simulink model "IRP"  (R2015a)
settings: Solver=ode1  StartTime=0.0  StopTime=Inf  FixedStep=0.001  RelTol=1e-3
PostLoadFcn:
  | , if any(exist('dsrtsu_mdlpostloadfcn', 'file') == [2, 3, 6]), try dsrtsu_mdlpostloadfcn('Execute', bdroot); catch fprintf('Error in PostLoadFcn (dsrtsu_mdlpostloadfcn) for model "%s":\n %s\n', bdroot, lasterr); end, end,
libraries: simulink x8, rtilibm x6, simulink_extras x6
(part 2 of 2)

== system IRP/P /Position 1/Filters 1 ==
  Sin && Cos : Inport
  Analog Butterworth LP Filter : Subsystem  mask(buttap){}
      mask help:
      | Analog Butterworth low pass filter.
      |
      | (Requires Signal Processing Toolbox)
      mask init:
      | [z,p,k]=buttap(@2); z=@1*z; p=@1*p; k=real(prod(-p)); [num,den]=zp2tf(z,p,k); w=logspace(log10(@1/10),log10(10*@1),20); h=freqs(num,den,w);
      mask Help: Butterworth low pass filter using MATLAB's butter command.
      mask Display: plot(20*log10(w),20*log10(abs(h)))
  Analog Butterworth LP Filter1 : Subsystem  mask(buttap){}
      mask help:
      | Analog Butterworth low pass filter.
      |
      | (Requires Signal Processing Toolbox)
      mask init:
      | [z,p,k]=buttap(@2); z=@1*z; p=@1*p; k=real(prod(-p)); [num,den]=zp2tf(z,p,k); w=logspace(log10(@1/10),log10(10*@1),20); h=freqs(num,den,w);
      mask Help: Butterworth low pass filter using MATLAB's butter command.
      mask Display: plot(20*log10(w),20*log10(abs(h)))
  Demux : Demux  Outputs=2
  Sin : Outport
  Cos : Outport  Port=2
  wires:
  Analog Butterworth LP Filter/1(Out1) -> Sin/1
  Analog Butterworth LP Filter1/1(Out1) -> Cos/1
  Sin && Cos/1 -> Demux/1
  Demux/1 -> Analog Butterworth LP Filter/1(In1)
  Demux/2 -> Analog Butterworth LP Filter1/1(In1)

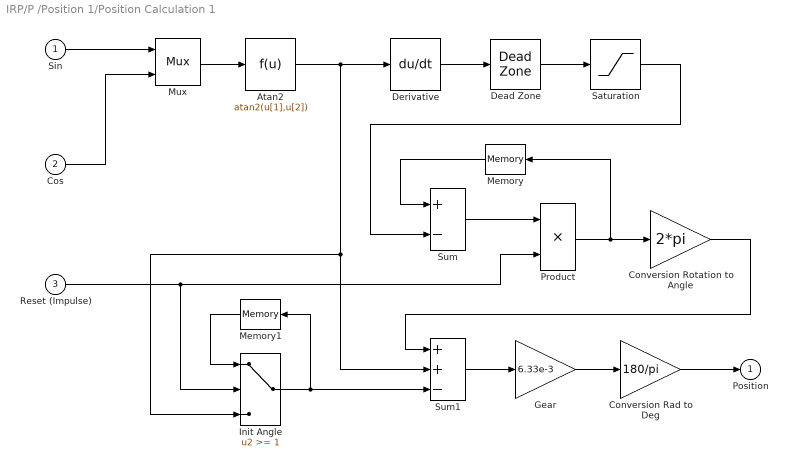
== system IRP/P /Position 1/Position Calculation 1 ==
  Sin : Inport
  Cos : Inport  Port=2
  Reset (Impulse) : Inport  Port=3
  Atan2 : Fcn  Expr=atan2(u[1],u[2])
  Conversion Rad to Deg : Gain  Gain=180/pi  SaturateOnIntegerOverflow=on  OutDataTypeStr=Inherit: Same as input  ParamDataTypeStr=Inherit: Same as input
  Conversion Rotation to Angle : Gain  Gain=2*pi  SaturateOnIntegerOverflow=on  OutDataTypeStr=Inherit: Same as input  ParamDataTypeStr=Inherit: Same as input
  Dead Zone : DeadZone  LowerValue=-5000  UpperValue=5000  SaturateOnIntegerOverflow=on
  Derivative : Derivative
  Gear : Gain  Gain=6.33e-3  SaturateOnIntegerOverflow=on  OutDataTypeStr=Inherit: Same as input  ParamDataTypeStr=Inherit: Same as input
  Init Angle : Switch  Threshold=1  SaturateOnIntegerOverflow=on  InputSameDT=on
  Memory : Memory
  Memory1 : Memory
  Mux : Mux  Inputs=2
  Product : Product  SaturateOnIntegerOverflow=on  RndMeth=Zero  InputSameDT=on  OutDataTypeStr=Inherit: Same as first input
  Saturation : Saturate  UpperLimit=1  LowerLimit=-1
  Sum : Sum  Inputs=+-  SaturateOnIntegerOverflow=on  InputSameDT=on  OutDataTypeStr=Inherit: Same as first input
  Sum1 : Sum  Inputs=++-  SaturateOnIntegerOverflow=on  InputSameDT=on  OutDataTypeStr=Inherit: Same as first input
  Position : Outport
  wires:
  Gear/1 -> Conversion Rad to Deg/1
  Sum1/1 -> Gear/1
  Sum/1 -> Product/1
  Dead Zone/1 -> Saturation/1
  Derivative/1 -> Dead Zone/1
  Mux/1 -> Atan2/1
  Sin/1 -> Mux/1
  Conversion Rad to Deg/1 -> Position/1
  Saturation/1 -> Sum/2
  Conversion Rotation to Angle/1 -> Sum1/1
  Reset (Impulse)/1 -> Product/2, Init Angle/2
  Atan2/1 -> Derivative/1, Sum1/2, Init Angle/3
  Cos/1 -> Mux/2
  Memory/1 -> Sum/1
  Product/1 -> Conversion Rotation to Angle/1, Memory/1
  Memory1/1 -> Init Angle/1
  Init Angle/1 -> Sum1/3, Memory1/1

== system IRP/P /Position 2/Filters 2 ==
  Sin && Cos : Inport
  Analog Butterworth LP Filter : Subsystem  mask(buttap){}
      mask help:
      | Analog Butterworth low pass filter.
      |
      | (Requires Signal Processing Toolbox)
      mask init:
      | [z,p,k]=buttap(@2); z=@1*z; p=@1*p; k=real(prod(-p)); [num,den]=zp2tf(z,p,k); w=logspace(log10(@1/10),log10(10*@1),20); h=freqs(num,den,w);
      mask Help: Butterworth low pass filter using MATLAB's butter command.
      mask Display: plot(20*log10(w),20*log10(abs(h)))
  Analog Butterworth LP Filter1 : Subsystem  mask(buttap){}
      mask help:
      | Analog Butterworth low pass filter.
      |
      | (Requires Signal Processing Toolbox)
      mask init:
      | [z,p,k]=buttap(@2); z=@1*z; p=@1*p; k=real(prod(-p)); [num,den]=zp2tf(z,p,k); w=logspace(log10(@1/10),log10(10*@1),20); h=freqs(num,den,w);
      mask Help: Butterworth low pass filter using MATLAB's butter command.
      mask Display: plot(20*log10(w),20*log10(abs(h)))
  Demux : Demux  Outputs=2
  Sin : Outport
  Cos : Outport  Port=2
  wires:
  Analog Butterworth LP Filter/1(Out1) -> Sin/1
  Analog Butterworth LP Filter1/1(Out1) -> Cos/1
  Sin && Cos/1 -> Demux/1
  Demux/1 -> Analog Butterworth LP Filter/1(In1)
  Demux/2 -> Analog Butterworth LP Filter1/1(In1)

== system IRP/P /Position 2/Position Calculation 2 ==
  Sin : Inport
  Cos : Inport  Port=2
  Reset (Impulse) : Inport  Port=3
  Atan2 : Fcn  Expr=atan2(u[1],u[2])
  Conversion Rad to Deg : Gain  Gain=180/pi  SaturateOnIntegerOverflow=on  OutDataTypeStr=Inherit: Same as input  ParamDataTypeStr=Inherit: Same as input
  Conversion Rotation to Angle : Gain  Gain=2*pi  SaturateOnIntegerOverflow=on  OutDataTypeStr=Inherit: Same as input  ParamDataTypeStr=Inherit: Same as input
  Dead Zone : DeadZone  LowerValue=-5000  UpperValue=5000  SaturateOnIntegerOverflow=on
  Derivative : Derivative
  Gear : Gain  Gain=6.37e-3  SaturateOnIntegerOverflow=on  OutDataTypeStr=Inherit: Same as input  ParamDataTypeStr=Inherit: Same as input
  Init Angle : Switch  Threshold=1  SaturateOnIntegerOverflow=on  InputSameDT=on
  Memory : Memory
  Memory1 : Memory
  Mux : Mux  Inputs=2
  Product : Product  SaturateOnIntegerOverflow=on  RndMeth=Zero  InputSameDT=on  OutDataTypeStr=Inherit: Same as first input
  Saturation : Saturate  UpperLimit=1  LowerLimit=-1
  Sum : Sum  Inputs=+-  SaturateOnIntegerOverflow=on  InputSameDT=on  OutDataTypeStr=Inherit: Same as first input
  Sum1 : Sum  Inputs=++-  SaturateOnIntegerOverflow=on  InputSameDT=on  OutDataTypeStr=Inherit: Same as first input
  Position : Outport
  wires:
  Gear/1 -> Conversion Rad to Deg/1
  Sum1/1 -> Gear/1
  Sum/1 -> Product/1
  Dead Zone/1 -> Saturation/1
  Derivative/1 -> Dead Zone/1
  Mux/1 -> Atan2/1
  Sin/1 -> Mux/1
  Conversion Rad to Deg/1 -> Position/1
  Saturation/1 -> Sum/2
  Conversion Rotation to Angle/1 -> Sum1/1
  Reset (Impulse)/1 -> Product/2, Init Angle/2
  Atan2/1 -> Derivative/1, Sum1/2, Init Angle/3
  Cos/1 -> Mux/2
  Memory/1 -> Sum/1
  Product/1 -> Conversion Rotation to Angle/1, Memory/1
  Memory1/1 -> Init Angle/1
  Init Angle/1 -> Sum1/3, Memory1/1

== system IRP/P /Position 3/Filters 3 ==
  Sin && Cos : Inport
  Analog Butterworth LP Filter : Subsystem  mask(buttap){}
      mask help:
      | Analog Butterworth low pass filter.
      |
      | (Requires Signal Processing Toolbox)
      mask init:
      | [z,p,k]=buttap(@2); z=@1*z; p=@1*p; k=real(prod(-p)); [num,den]=zp2tf(z,p,k); w=logspace(log10(@1/10),log10(10*@1),20); h=freqs(num,den,w);
      mask Help: Butterworth low pass filter using MATLAB's butter command.
      mask Display: plot(20*log10(w),20*log10(abs(h)))
  Analog Butterworth LP Filter1 : Subsystem  mask(buttap){}
      mask help:
      | Analog Butterworth low pass filter.
      |
      | (Requires Signal Processing Toolbox)
      mask init:
      | [z,p,k]=buttap(@2); z=@1*z; p=@1*p; k=real(prod(-p)); [num,den]=zp2tf(z,p,k); w=logspace(log10(@1/10),log10(10*@1),20); h=freqs(num,den,w);
      mask Help: Butterworth low pass filter using MATLAB's butter command.
      mask Display: plot(20*log10(w),20*log10(abs(h)))
  Demux : Demux  Outputs=2
  Sin : Outport
  Cos : Outport  Port=2
  wires:
  Analog Butterworth LP Filter/1(Out1) -> Sin/1
  Analog Butterworth LP Filter1/1(Out1) -> Cos/1
  Sin && Cos/1 -> Demux/1
  Demux/1 -> Analog Butterworth LP Filter/1(In1)
  Demux/2 -> Analog Butterworth LP Filter1/1(In1)

== system IRP/P /Position 3/Position Calculation 3 ==
  Sin : Inport
  Cos : Inport  Port=2
  Reset (Impulse) : Inport  Port=3
  Atan2 : Fcn  Expr=atan2(u[1],u[2])
  Conversion Rad to Deg : Gain  Gain=180/pi  SaturateOnIntegerOverflow=on  OutDataTypeStr=Inherit: Same as input  ParamDataTypeStr=Inherit: Same as input
  Conversion Rotation to Angle : Gain  Gain=2*pi  SaturateOnIntegerOverflow=on  OutDataTypeStr=Inherit: Same as input  ParamDataTypeStr=Inherit: Same as input
  Dead Zone : DeadZone  LowerValue=-5000  UpperValue=5000  SaturateOnIntegerOverflow=on
  Derivative : Derivative
  Gear : Gain  Gain=6.33e-3  SaturateOnIntegerOverflow=on  OutDataTypeStr=Inherit: Same as input  ParamDataTypeStr=Inherit: Same as input
  Init Angle : Switch  Threshold=1  SaturateOnIntegerOverflow=on  InputSameDT=on
  Memory : Memory
  Memory1 : Memory
  Mux : Mux  Inputs=2
  Product : Product  SaturateOnIntegerOverflow=on  RndMeth=Zero  InputSameDT=on  OutDataTypeStr=Inherit: Same as first input
  Saturation : Saturate  UpperLimit=1  LowerLimit=-1
  Sum : Sum  Inputs=+-  SaturateOnIntegerOverflow=on  InputSameDT=on  OutDataTypeStr=Inherit: Same as first input
  Sum1 : Sum  Inputs=++-  SaturateOnIntegerOverflow=on  InputSameDT=on  OutDataTypeStr=Inherit: Same as first input
  Position : Outport
  wires:
  Gear/1 -> Conversion Rad to Deg/1
  Sum1/1 -> Gear/1
  Sum/1 -> Product/1
  Dead Zone/1 -> Saturation/1
  Derivative/1 -> Dead Zone/1
  Mux/1 -> Atan2/1
  Sin/1 -> Mux/1
  Conversion Rad to Deg/1 -> Position/1
  Saturation/1 -> Sum/2
  Conversion Rotation to Angle/1 -> Sum1/1
  Reset (Impulse)/1 -> Product/2, Init Angle/2
  Atan2/1 -> Derivative/1, Sum1/2, Init Angle/3
  Cos/1 -> Mux/2
  Memory/1 -> Sum/1
  Product/1 -> Conversion Rotation to Angle/1, Memory/1
  Memory1/1 -> Init Angle/1
  Init Angle/1 -> Sum1/3, Memory1/1

== system IRP/P /Position 4/Filters 4 ==
  Sin && Cos : Inport
  Analog Butterworth LP Filter : Subsystem  mask(buttap){}
      mask help:
      | Analog Butterworth low pass filter.
      |
      | (Requires Signal Processing Toolbox)
      mask init:
      | [z,p,k]=buttap(@2); z=@1*z; p=@1*p; k=real(prod(-p)); [num,den]=zp2tf(z,p,k); w=logspace(log10(@1/10),log10(10*@1),20); h=freqs(num,den,w);
      mask Help: Butterworth low pass filter using MATLAB's butter command.
      mask Display: plot(20*log10(w),20*log10(abs(h)))
  Analog Butterworth LP Filter1 : Subsystem  mask(buttap){}
      mask help:
      | Analog Butterworth low pass filter.
      |
      | (Requires Signal Processing Toolbox)
      mask init:
      | [z,p,k]=buttap(@2); z=@1*z; p=@1*p; k=real(prod(-p)); [num,den]=zp2tf(z,p,k); w=logspace(log10(@1/10),log10(10*@1),20); h=freqs(num,den,w);
      mask Help: Butterworth low pass filter using MATLAB's butter command.
      mask Display: plot(20*log10(w),20*log10(abs(h)))
  Demux : Demux  Outputs=2
  Sin : Outport
  Cos : Outport  Port=2
  wires:
  Demux/2 -> Analog Butterworth LP Filter1/1(In1)
  Demux/1 -> Analog Butterworth LP Filter/1(In1)
  Sin && Cos/1 -> Demux/1
  Analog Butterworth LP Filter1/1(Out1) -> Cos/1
  Analog Butterworth LP Filter/1(Out1) -> Sin/1

== system IRP/P /Position 4/Position Calculation 4 ==
  Sin : Inport
  Cos : Inport  Port=2
  Reset (Impulse) : Inport  Port=3
  Atan2 : Fcn  Expr=atan2(u[1],u[2])
  Conversion Rad to Deg : Gain  Gain=180/pi  SaturateOnIntegerOverflow=on  OutDataTypeStr=Inherit: Same as input  ParamDataTypeStr=Inherit: Same as input
  Conversion Rotation to Angle : Gain  Gain=2*pi  SaturateOnIntegerOverflow=on  OutDataTypeStr=Inherit: Same as input  ParamDataTypeStr=Inherit: Same as input
  Dead Zone : DeadZone  LowerValue=-5000  UpperValue=5000  SaturateOnIntegerOverflow=on
  Derivative : Derivative
  Gear : Gain  Gain=7.87e-3  SaturateOnIntegerOverflow=on  OutDataTypeStr=Inherit: Same as input  ParamDataTypeStr=Inherit: Same as input
  Init Angle : Switch  Threshold=1  SaturateOnIntegerOverflow=on  InputSameDT=on
  Memory : Memory
  Memory1 : Memory
  Mux : Mux  Inputs=2
  Product : Product  SaturateOnIntegerOverflow=on  RndMeth=Zero  InputSameDT=on  OutDataTypeStr=Inherit: Same as first input
  Saturation : Saturate  UpperLimit=1  LowerLimit=-1
  Sum : Sum  Inputs=+-  SaturateOnIntegerOverflow=on  InputSameDT=on  OutDataTypeStr=Inherit: Same as first input
  Sum1 : Sum  Inputs=++-  SaturateOnIntegerOverflow=on  InputSameDT=on  OutDataTypeStr=Inherit: Same as first input
  Position : Outport
  wires:
  Init Angle/1 -> Memory1/1, Sum1/3
  Memory1/1 -> Init Angle/1
  Product/1 -> Memory/1, Conversion Rotation to Angle/1
  Memory/1 -> Sum/1
  Cos/1 -> Mux/2
  Atan2/1 -> Init Angle/3, Sum1/2, Derivative/1
  Reset (Impulse)/1 -> Init Angle/2, Product/2
  Conversion Rotation to Angle/1 -> Sum1/1
  Saturation/1 -> Sum/2
  Conversion Rad to Deg/1 -> Position/1
  Sin/1 -> Mux/1
  Mux/1 -> Atan2/1
  Derivative/1 -> Dead Zone/1
  Dead Zone/1 -> Saturation/1
  Sum/1 -> Product/1
  Sum1/1 -> Gear/1
  Gear/1 -> Conversion Rad to Deg/1

== system IRP/P /Position 5/Filters 5 ==
  Sin && Cos : Inport
  Analog Butterworth LP Filter : Subsystem  mask(buttap){}
      mask help:
      | Analog Butterworth low pass filter.
      |
      | (Requires Signal Processing Toolbox)
      mask init:
      | [z,p,k]=buttap(@2); z=@1*z; p=@1*p; k=real(prod(-p)); [num,den]=zp2tf(z,p,k); w=logspace(log10(@1/10),log10(10*@1),20); h=freqs(num,den,w);
      mask Help: Butterworth low pass filter using MATLAB's butter command.
      mask Display: plot(20*log10(w),20*log10(abs(h)))
  Analog Butterworth LP Filter1 : Subsystem  mask(buttap){}
      mask help:
      | Analog Butterworth low pass filter.
      |
      | (Requires Signal Processing Toolbox)
      mask init:
      | [z,p,k]=buttap(@2); z=@1*z; p=@1*p; k=real(prod(-p)); [num,den]=zp2tf(z,p,k); w=logspace(log10(@1/10),log10(10*@1),20); h=freqs(num,den,w);
      mask Help: Butterworth low pass filter using MATLAB's butter command.
      mask Display: plot(20*log10(w),20*log10(abs(h)))
  Demux : Demux  Outputs=2
  Sin : Outport
  Cos : Outport  Port=2
  wires:
  Demux/2 -> Analog Butterworth LP Filter1/1(In1)
  Demux/1 -> Analog Butterworth LP Filter/1(In1)
  Sin && Cos/1 -> Demux/1
  Analog Butterworth LP Filter1/1(Out1) -> Cos/1
  Analog Butterworth LP Filter/1(Out1) -> Sin/1

== system IRP/P /Position 5/Position Calculation 5 ==
  Sin : Inport
  Cos : Inport  Port=2
  Reset (Impulse) : Inport  Port=3
  Atan2 : Fcn  Expr=atan2(u[1],u[2])
  Conversion Rad to Deg : Gain  Gain=180/pi  SaturateOnIntegerOverflow=on  OutDataTypeStr=Inherit: Same as input  ParamDataTypeStr=Inherit: Same as input
  Conversion Rotation to Angle : Gain  Gain=2*pi  SaturateOnIntegerOverflow=on  OutDataTypeStr=Inherit: Same as input  ParamDataTypeStr=Inherit: Same as input
  Dead Zone : DeadZone  LowerValue=-5000  UpperValue=5000  SaturateOnIntegerOverflow=on
  Derivative : Derivative
  Gear : Gain  Gain=1.32e-2  SaturateOnIntegerOverflow=on  OutDataTypeStr=Inherit: Same as input  ParamDataTypeStr=Inherit: Same as input
  Init Angle : Switch  Threshold=1  SaturateOnIntegerOverflow=on  InputSameDT=on
  Memory : Memory
  Memory1 : Memory
  Mux : Mux  Inputs=2
  Product : Product  SaturateOnIntegerOverflow=on  RndMeth=Zero  InputSameDT=on  OutDataTypeStr=Inherit: Same as first input
  Saturation : Saturate  UpperLimit=1  LowerLimit=-1
  Sum : Sum  Inputs=+-  SaturateOnIntegerOverflow=on  InputSameDT=on  OutDataTypeStr=Inherit: Same as first input
  Sum1 : Sum  Inputs=++-  SaturateOnIntegerOverflow=on  InputSameDT=on  OutDataTypeStr=Inherit: Same as first input
  Position : Outport
  wires:
  Init Angle/1 -> Memory1/1, Sum1/3
  Memory1/1 -> Init Angle/1
  Product/1 -> Memory/1, Conversion Rotation to Angle/1
  Memory/1 -> Sum/1
  Cos/1 -> Mux/2
  Atan2/1 -> Init Angle/3, Sum1/2, Derivative/1
  Reset (Impulse)/1 -> Init Angle/2, Product/2
  Conversion Rotation to Angle/1 -> Sum1/1
  Saturation/1 -> Sum/2
  Conversion Rad to Deg/1 -> Position/1
  Sin/1 -> Mux/1
  Mux/1 -> Atan2/1
  Derivative/1 -> Dead Zone/1
  Dead Zone/1 -> Saturation/1
  Sum/1 -> Product/1
  Sum1/1 -> Gear/1
  Gear/1 -> Conversion Rad to Deg/1

== system IRP/RTI Data/RTI Data Store/RTI Data Store ==
  RTI Data Store : Subsystem  mask(RTI_DATA_STORE){}
      mask help:
      | RTI Data Store Block. This block is used by RTI to store internal model dependent data. Deleting this block will result in data loss.
      |
      | NEVER DELETE, COPY, OR MODIFY THIS BLOCK!
      mask Help:
      | RTI Data Store Block. This block is used by RTI to store internal model dependent data. Deleting this block will result in data loss.
      | 
      | NEVER DELETE, COPY, OR MODIFY THIS BLOCK!
      mask Display: text(0.5, 0.5, ' ', 'HorizontalAlignment', 'center');

== system IRP/Const/Subsystem/Position 1/Filters 1 ==
  Sin && Cos : Inport
  Analog Butterworth LP Filter : Subsystem  mask(buttap){}
      mask help:
      | Analog Butterworth low pass filter.
      |
      | (Requires Signal Processing Toolbox)
      mask init:
      | [z,p,k]=buttap(@2); z=@1*z; p=@1*p; k=real(prod(-p)); [num,den]=zp2tf(z,p,k); w=logspace(log10(@1/10),log10(10*@1),20); h=freqs(num,den,w);
      mask Help: Butterworth low pass filter using MATLAB's butter command.
      mask Display: plot(20*log10(w),20*log10(abs(h)))
  Analog Butterworth LP Filter1 : Subsystem  mask(buttap){}
      mask help:
      | Analog Butterworth low pass filter.
      |
      | (Requires Signal Processing Toolbox)
      mask init:
      | [z,p,k]=buttap(@2); z=@1*z; p=@1*p; k=real(prod(-p)); [num,den]=zp2tf(z,p,k); w=logspace(log10(@1/10),log10(10*@1),20); h=freqs(num,den,w);
      mask Help: Butterworth low pass filter using MATLAB's butter command.
      mask Display: plot(20*log10(w),20*log10(abs(h)))
  Demux : Demux  Outputs=2
  Sin : Outport
  Cos : Outport  Port=2
  wires:
  Analog Butterworth LP Filter/1(Out1) -> Sin/1
  Analog Butterworth LP Filter1/1(Out1) -> Cos/1
  Sin && Cos/1 -> Demux/1
  Demux/1 -> Analog Butterworth LP Filter/1(In1)
  Demux/2 -> Analog Butterworth LP Filter1/1(In1)

== system IRP/Const/Subsystem/Position 1/Position Calculation 1 ==
  Sin : Inport
  Cos : Inport  Port=2
  Reset (Impulse) : Inport  Port=3
  Atan2 : Fcn  Expr=atan2(u[1],u[2])
  Conversion Rad to Deg : Gain  Gain=180/pi  SaturateOnIntegerOverflow=on  OutDataTypeStr=Inherit: Same as input  ParamDataTypeStr=Inherit: Same as input
  Conversion Rotation to Angle : Gain  Gain=2*pi  SaturateOnIntegerOverflow=on  OutDataTypeStr=Inherit: Same as input  ParamDataTypeStr=Inherit: Same as input
  Dead Zone : DeadZone  LowerValue=-5000  UpperValue=5000  SaturateOnIntegerOverflow=on
  Derivative : Derivative
  Gear : Gain  Gain=6.33e-3  SaturateOnIntegerOverflow=on  OutDataTypeStr=Inherit: Same as input  ParamDataTypeStr=Inherit: Same as input
  Init Angle : Switch  Threshold=1  SaturateOnIntegerOverflow=on  InputSameDT=on
  Memory : Memory
  Memory1 : Memory
  Mux : Mux  Inputs=2
  Product : Product  SaturateOnIntegerOverflow=on  RndMeth=Zero  InputSameDT=on  OutDataTypeStr=Inherit: Same as first input
  Saturation : Saturate  UpperLimit=1  LowerLimit=-1
  Sum : Sum  Inputs=+-  SaturateOnIntegerOverflow=on  InputSameDT=on  OutDataTypeStr=Inherit: Same as first input
  Sum1 : Sum  Inputs=++-  SaturateOnIntegerOverflow=on  InputSameDT=on  OutDataTypeStr=Inherit: Same as first input
  Position : Outport
  wires:
  Gear/1 -> Conversion Rad to Deg/1
  Sum1/1 -> Gear/1
  Sum/1 -> Product/1
  Dead Zone/1 -> Saturation/1
  Derivative/1 -> Dead Zone/1
  Mux/1 -> Atan2/1
  Sin/1 -> Mux/1
  Conversion Rad to Deg/1 -> Position/1
  Saturation/1 -> Sum/2
  Conversion Rotation to Angle/1 -> Sum1/1
  Reset (Impulse)/1 -> Product/2, Init Angle/2
  Atan2/1 -> Derivative/1, Sum1/2, Init Angle/3
  Cos/1 -> Mux/2
  Memory/1 -> Sum/1
  Product/1 -> Conversion Rotation to Angle/1, Memory/1
  Memory1/1 -> Init Angle/1
  Init Angle/1 -> Sum1/3, Memory1/1

== system IRP/Const/Subsystem/Position 2/Filters 2 ==
  Sin && Cos : Inport
  Analog Butterworth LP Filter : Subsystem  mask(buttap){}
      mask help:
      | Analog Butterworth low pass filter.
      |
      | (Requires Signal Processing Toolbox)
      mask init:
      | [z,p,k]=buttap(@2); z=@1*z; p=@1*p; k=real(prod(-p)); [num,den]=zp2tf(z,p,k); w=logspace(log10(@1/10),log10(10*@1),20); h=freqs(num,den,w);
      mask Help: Butterworth low pass filter using MATLAB's butter command.
      mask Display: plot(20*log10(w),20*log10(abs(h)))
  Analog Butterworth LP Filter1 : Subsystem  mask(buttap){}
      mask help:
      | Analog Butterworth low pass filter.
      |
      | (Requires Signal Processing Toolbox)
      mask init:
      | [z,p,k]=buttap(@2); z=@1*z; p=@1*p; k=real(prod(-p)); [num,den]=zp2tf(z,p,k); w=logspace(log10(@1/10),log10(10*@1),20); h=freqs(num,den,w);
      mask Help: Butterworth low pass filter using MATLAB's butter command.
      mask Display: plot(20*log10(w),20*log10(abs(h)))
  Demux : Demux  Outputs=2
  Sin : Outport
  Cos : Outport  Port=2
  wires:
  Analog Butterworth LP Filter/1(Out1) -> Sin/1
  Analog Butterworth LP Filter1/1(Out1) -> Cos/1
  Sin && Cos/1 -> Demux/1
  Demux/1 -> Analog Butterworth LP Filter/1(In1)
  Demux/2 -> Analog Butterworth LP Filter1/1(In1)

== system IRP/Const/Subsystem/Position 2/Position Calculation 2 ==
  Sin : Inport
  Cos : Inport  Port=2
  Reset (Impulse) : Inport  Port=3
  Atan2 : Fcn  Expr=atan2(u[1],u[2])
  Conversion Rad to Deg : Gain  Gain=180/pi  SaturateOnIntegerOverflow=on  OutDataTypeStr=Inherit: Same as input  ParamDataTypeStr=Inherit: Same as input
  Conversion Rotation to Angle : Gain  Gain=2*pi  SaturateOnIntegerOverflow=on  OutDataTypeStr=Inherit: Same as input  ParamDataTypeStr=Inherit: Same as input
  Dead Zone : DeadZone  LowerValue=-5000  UpperValue=5000  SaturateOnIntegerOverflow=on
  Derivative : Derivative
  Gear : Gain  Gain=6.37e-3  SaturateOnIntegerOverflow=on  OutDataTypeStr=Inherit: Same as input  ParamDataTypeStr=Inherit: Same as input
  Init Angle : Switch  Threshold=1  SaturateOnIntegerOverflow=on  InputSameDT=on
  Memory : Memory
  Memory1 : Memory
  Mux : Mux  Inputs=2
  Product : Product  SaturateOnIntegerOverflow=on  RndMeth=Zero  InputSameDT=on  OutDataTypeStr=Inherit: Same as first input
  Saturation : Saturate  UpperLimit=1  LowerLimit=-1
  Sum : Sum  Inputs=+-  SaturateOnIntegerOverflow=on  InputSameDT=on  OutDataTypeStr=Inherit: Same as first input
  Sum1 : Sum  Inputs=++-  SaturateOnIntegerOverflow=on  InputSameDT=on  OutDataTypeStr=Inherit: Same as first input
  Position : Outport
  wires:
  Gear/1 -> Conversion Rad to Deg/1
  Sum1/1 -> Gear/1
  Sum/1 -> Product/1
  Dead Zone/1 -> Saturation/1
  Derivative/1 -> Dead Zone/1
  Mux/1 -> Atan2/1
  Sin/1 -> Mux/1
  Conversion Rad to Deg/1 -> Position/1
  Saturation/1 -> Sum/2
  Conversion Rotation to Angle/1 -> Sum1/1
  Reset (Impulse)/1 -> Product/2, Init Angle/2
  Atan2/1 -> Derivative/1, Sum1/2, Init Angle/3
  Cos/1 -> Mux/2
  Memory/1 -> Sum/1
  Product/1 -> Conversion Rotation to Angle/1, Memory/1
  Memory1/1 -> Init Angle/1
  Init Angle/1 -> Sum1/3, Memory1/1

== system IRP/Const/Subsystem/Position 3/Filters 3 ==
  Sin && Cos : Inport
  Analog Butterworth LP Filter : Subsystem  mask(buttap){}
      mask help:
      | Analog Butterworth low pass filter.
      |
      | (Requires Signal Processing Toolbox)
      mask init:
      | [z,p,k]=buttap(@2); z=@1*z; p=@1*p; k=real(prod(-p)); [num,den]=zp2tf(z,p,k); w=logspace(log10(@1/10),log10(10*@1),20); h=freqs(num,den,w);
      mask Help: Butterworth low pass filter using MATLAB's butter command.
      mask Display: plot(20*log10(w),20*log10(abs(h)))
  Analog Butterworth LP Filter1 : Subsystem  mask(buttap){}
      mask help:
      | Analog Butterworth low pass filter.
      |
      | (Requires Signal Processing Toolbox)
      mask init:
      | [z,p,k]=buttap(@2); z=@1*z; p=@1*p; k=real(prod(-p)); [num,den]=zp2tf(z,p,k); w=logspace(log10(@1/10),log10(10*@1),20); h=freqs(num,den,w);
      mask Help: Butterworth low pass filter using MATLAB's butter command.
      mask Display: plot(20*log10(w),20*log10(abs(h)))
  Demux : Demux  Outputs=2
  Sin : Outport
  Cos : Outport  Port=2
  wires:
  Analog Butterworth LP Filter/1(Out1) -> Sin/1
  Analog Butterworth LP Filter1/1(Out1) -> Cos/1
  Sin && Cos/1 -> Demux/1
  Demux/1 -> Analog Butterworth LP Filter/1(In1)
  Demux/2 -> Analog Butterworth LP Filter1/1(In1)

== system IRP/Const/Subsystem/Position 3/Position Calculation 3 ==
  Sin : Inport
  Cos : Inport  Port=2
  Reset (Impulse) : Inport  Port=3
  Atan2 : Fcn  Expr=atan2(u[1],u[2])
  Conversion Rad to Deg : Gain  Gain=180/pi  SaturateOnIntegerOverflow=on  OutDataTypeStr=Inherit: Same as input  ParamDataTypeStr=Inherit: Same as input
  Conversion Rotation to Angle : Gain  Gain=2*pi  SaturateOnIntegerOverflow=on  OutDataTypeStr=Inherit: Same as input  ParamDataTypeStr=Inherit: Same as input
  Dead Zone : DeadZone  LowerValue=-5000  UpperValue=5000  SaturateOnIntegerOverflow=on
  Derivative : Derivative
  Gear : Gain  Gain=6.33e-3  SaturateOnIntegerOverflow=on  OutDataTypeStr=Inherit: Same as input  ParamDataTypeStr=Inherit: Same as input
  Init Angle : Switch  Threshold=1  SaturateOnIntegerOverflow=on  InputSameDT=on
  Memory : Memory
  Memory1 : Memory
  Mux : Mux  Inputs=2
  Product : Product  SaturateOnIntegerOverflow=on  RndMeth=Zero  InputSameDT=on  OutDataTypeStr=Inherit: Same as first input
  Saturation : Saturate  UpperLimit=1  LowerLimit=-1
  Sum : Sum  Inputs=+-  SaturateOnIntegerOverflow=on  InputSameDT=on  OutDataTypeStr=Inherit: Same as first input
  Sum1 : Sum  Inputs=++-  SaturateOnIntegerOverflow=on  InputSameDT=on  OutDataTypeStr=Inherit: Same as first input
  Position : Outport
  wires:
  Gear/1 -> Conversion Rad to Deg/1
  Sum1/1 -> Gear/1
  Sum/1 -> Product/1
  Dead Zone/1 -> Saturation/1
  Derivative/1 -> Dead Zone/1
  Mux/1 -> Atan2/1
  Sin/1 -> Mux/1
  Conversion Rad to Deg/1 -> Position/1
  Saturation/1 -> Sum/2
  Conversion Rotation to Angle/1 -> Sum1/1
  Reset (Impulse)/1 -> Product/2, Init Angle/2
  Atan2/1 -> Derivative/1, Sum1/2, Init Angle/3
  Cos/1 -> Mux/2
  Memory/1 -> Sum/1
  Product/1 -> Conversion Rotation to Angle/1, Memory/1
  Memory1/1 -> Init Angle/1
  Init Angle/1 -> Sum1/3, Memory1/1

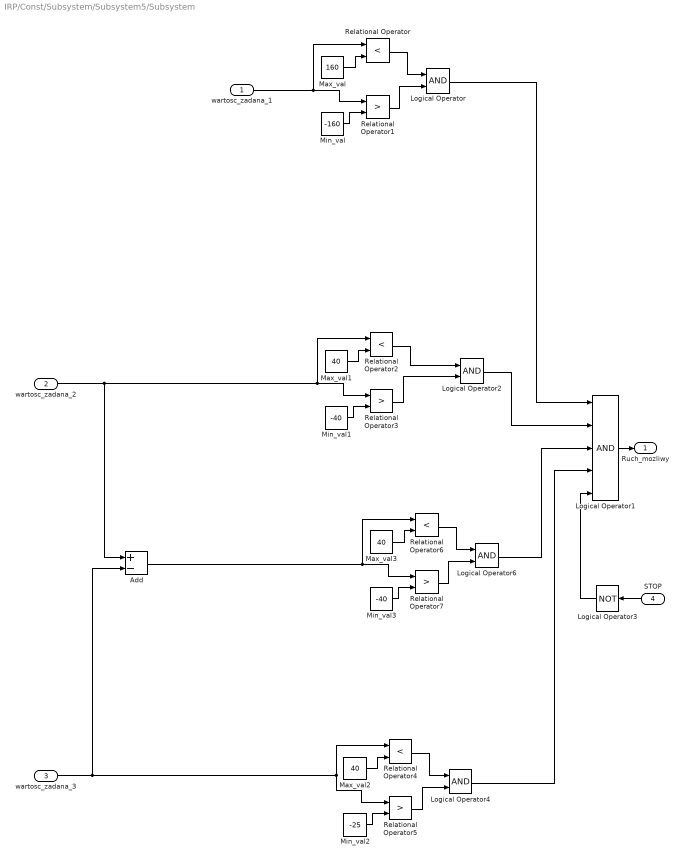
== system IRP/Const/Subsystem/Subsystem5/Subsystem ==
  wartosc_zadana_1 : Inport
  wartosc_zadana_2 : Inport  Port=2
  wartosc_zadana_3 : Inport  Port=3
  STOP : Inport  Port=4
  Add : Sum  Inputs=+-
  Logical Operator{,2,4,6} (4 alike) : Logic  AllPortsSameDT=off
  Logical Operator1 : Logic  Inputs=5  AllPortsSameDT=off
  Logical Operator3 : Logic  Operator=NOT  AllPortsSameDT=off
  Max_val : Constant  Value=160
  Max_val1 : Constant  Value=40
  Max_val2 : Constant  Value=40
  Max_val3 : Constant  Value=40
  Min_val : Constant  Value=-160
  Min_val1 : Constant  Value=-40
  Min_val2 : Constant  Value=-25
  Min_val3 : Constant  Value=-40
  Relational Operator{,2,4,6} (4 alike) : RelationalOperator  Operator=<  OutDataTypeStr=boolean
  Relational Operator{1,3,5,7} (4 alike) : RelationalOperator  Operator=>  OutDataTypeStr=boolean
  Ruch_mozliwy : Outport
  wires:
  wartosc_zadana_3/1 -> Add/2, Relational Operator5/1, Relational Operator4/1
  Max_val1/1 -> Relational Operator2/2
  Relational Operator4/1 -> Logical Operator4/1
  Relational Operator3/1 -> Logical Operator2/2
  Relational Operator2/1 -> Logical Operator2/1
  Min_val1/1 -> Relational Operator3/2
  wartosc_zadana_2/1 -> Add/1, Relational Operator3/1, Relational Operator2/1
  Relational Operator5/1 -> Logical Operator4/2
  Min_val3/1 -> Relational Operator7/2
  Relational Operator6/1 -> Logical Operator6/1
  Max_val3/1 -> Relational Operator6/2
  Relational Operator7/1 -> Logical Operator6/2
  Logical Operator4/1 -> Logical Operator1/4
  Add/1 -> Relational Operator7/1, Relational Operator6/1
  Logical Operator/1 -> Logical Operator1/1
  Logical Operator6/1 -> Logical Operator1/3
  Logical Operator2/1 -> Logical Operator1/2
  STOP/1 -> Logical Operator3/1
  Logical Operator1/1 -> Ruch_mozliwy/1
  Logical Operator3/1 -> Logical Operator1/5
  Max_val2/1 -> Relational Operator4/2
  Min_val2/1 -> Relational Operator5/2
  Max_val/1 -> Relational Operator/2
  Min_val/1 -> Relational Operator1/2
  wartosc_zadana_1/1 -> Relational Operator1/1, Relational Operator/1
  Relational Operator1/1 -> Logical Operator/2
  Relational Operator/1 -> Logical Operator/1

== system IRP/Const/Subsystem/serwo_1/Subsystem ==
  rozpoczecie_bazowania : Inport
  sygnal_bazowy : Inport  Port=2
  Data Type Conversion : DataTypeConversion  OutDataTypeStr=boolean
  Data Type Conversion1 : DataTypeConversion  OutDataTypeStr=boolean
  Detect Fall Nonpositive : simulink/Logic and Bit Operations/Detect Fall Nonpositive  vinit=0  InputProcessing=Inherited  OutDataTypeStr=boolean
  S-R Flip-Flop : simulink_extras/Flip Flops/S-R Flip-Flop  initial_condition=0
  Terminator : Terminator
  trwa_bazowanie : Outport
  zerowanie : Outport  Port=2
  wires:
  S-R Flip-Flop/1 -> trwa_bazowanie/1, Detect Fall Nonpositive/1
  S-R Flip-Flop/2 -> Terminator/1
  sygnal_bazowy/1 -> Data Type Conversion1/1
  Data Type Conversion/1 -> S-R Flip-Flop/1
  Data Type Conversion1/1 -> S-R Flip-Flop/2
  Detect Fall Nonpositive/1 -> zerowanie/1
  rozpoczecie_bazowania/1 -> Data Type Conversion/1

== system IRP/Const/Subsystem/serwo_1/Subsystem1 ==
  biezacy uchyb : Inport
  max uchyb : Inport  Port=2
  Divide : Product  Inputs=*/
  Saturation1 : Saturate  UpperLimit=1  LowerLimit=0.001
  wspolczynnik : Outport
  wires:
  max uchyb/1 -> Divide/2
  biezacy uchyb/1 -> Divide/1
  Divide/1 -> Saturation1/1
  Saturation1/1 -> wspolczynnik/1

== system IRP/Const/Subsystem/serwo_2/Subsystem ==
  rozpoczecie_bazowania : Inport
  sygnal_bazowy : Inport  Port=2
  Data Type Conversion : DataTypeConversion  OutDataTypeStr=boolean
  Data Type Conversion1 : DataTypeConversion  OutDataTypeStr=boolean
  Detect Fall Nonpositive : simulink/Logic and Bit Operations/Detect Fall Nonpositive  vinit=0  InputProcessing=Inherited  OutDataTypeStr=boolean
  S-R Flip-Flop : simulink_extras/Flip Flops/S-R Flip-Flop  initial_condition=0
  Terminator : Terminator
  trwa_bazowanie : Outport
  zerowanie : Outport  Port=2
  wires:
  S-R Flip-Flop/1 -> trwa_bazowanie/1, Detect Fall Nonpositive/1
  S-R Flip-Flop/2 -> Terminator/1
  sygnal_bazowy/1 -> Data Type Conversion1/1
  Data Type Conversion/1 -> S-R Flip-Flop/1
  Data Type Conversion1/1 -> S-R Flip-Flop/2
  Detect Fall Nonpositive/1 -> zerowanie/1
  rozpoczecie_bazowania/1 -> Data Type Conversion/1

== system IRP/Const/Subsystem/serwo_2/Subsystem1 ==
  biezacy uchyb : Inport
  max uchyb : Inport  Port=2
  Divide : Product  Inputs=*/
  Saturation1 : Saturate  UpperLimit=1  LowerLimit=0.001
  wspolczynnik : Outport
  wires:
  max uchyb/1 -> Divide/2
  biezacy uchyb/1 -> Divide/1
  Divide/1 -> Saturation1/1
  Saturation1/1 -> wspolczynnik/1

== system IRP/Const/Subsystem/serwo_3/Subsystem ==
  rozpoczecie_bazowania : Inport
  sygnal_bazowy : Inport  Port=2
  Data Type Conversion : DataTypeConversion  OutDataTypeStr=boolean
  Data Type Conversion1 : DataTypeConversion  OutDataTypeStr=boolean
  Detect Fall Nonpositive : simulink/Logic and Bit Operations/Detect Fall Nonpositive  vinit=0  InputProcessing=Inherited  OutDataTypeStr=boolean
  S-R Flip-Flop : simulink_extras/Flip Flops/S-R Flip-Flop  initial_condition=0
  Terminator : Terminator
  trwa_bazowanie : Outport
  zerowanie : Outport  Port=2
  wires:
  S-R Flip-Flop/1 -> trwa_bazowanie/1, Detect Fall Nonpositive/1
  S-R Flip-Flop/2 -> Terminator/1
  sygnal_bazowy/1 -> Data Type Conversion1/1
  Data Type Conversion/1 -> S-R Flip-Flop/1
  Data Type Conversion1/1 -> S-R Flip-Flop/2
  Detect Fall Nonpositive/1 -> zerowanie/1
  rozpoczecie_bazowania/1 -> Data Type Conversion/1

== system IRP/Const/Subsystem/serwo_3/Subsystem1 ==
  biezacy uchyb : Inport
  max uchyb : Inport  Port=2
  Divide : Product  Inputs=*/
  Saturation1 : Saturate  UpperLimit=1  LowerLimit=0.001
  wspolczynnik : Outport
  wires:
  max uchyb/1 -> Divide/2
  biezacy uchyb/1 -> Divide/1
  Divide/1 -> Saturation1/1
  Saturation1/1 -> wspolczynnik/1

== system IRP/Const/Subsystem/serwo_4_5/Position 4 ==
  Sin && Cos4 : Inport
  Reset 4 : Inport  Port=2
  Filters 4 : Subsystem
  Position Calculation 4 : Subsystem
  Out1 : Outport
  wires:
  Filters 4/1(Sin) -> Position Calculation 4/1(Sin)
  Filters 4/2(Cos) -> Position Calculation 4/2(Cos)
  Sin && Cos4/1 -> Filters 4/1(Sin && Cos)
  Reset 4/1 -> Position Calculation 4/3(Reset (Impulse))
  Position Calculation 4/1(Position) -> Out1/1

== system IRP/Const/Subsystem/serwo_4_5/Position 5 ==
  Sin && Cos5 : Inport
  Reset 5 : Inport  Port=2
  Filters 5 : Subsystem
  Position Calculation 5 : Subsystem
  Out1 : Outport
  wires:
  Filters 5/1(Sin) -> Position Calculation 5/1(Sin)
  Filters 5/2(Cos) -> Position Calculation 5/2(Cos)
  Sin && Cos5/1 -> Filters 5/1(Sin && Cos)
  Reset 5/1 -> Position Calculation 5/3(Reset (Impulse))
  Position Calculation 5/1(Position) -> Out1/1

== system IRP/Const/Subsystem/serwo_4_5/serwo_4 ==
  wartosc_zad : Inport
  pomiar_poloz : Inport  Port=2
  Gain : Gain  Gain=0.5
  Rate Limiter : RateLimiter  RisingSlewLimit=50  FallingSlewLimit=-50  SampleTimeMode=inherited
  Saturation : Saturate  UpperLimit=3  LowerLimit=-3
  Sum : Sum  Inputs=|+-
  ograniczenie sygnalu : Gain  Gain=0.1
  dac_out : Outport
  wires:
  pomiar_poloz/1 -> Sum/2
  wartosc_zad/1 -> Sum/1
  Saturation/1 -> Rate Limiter/1
  Gain/1 -> Saturation/1
  Sum/1 -> Gain/1
  Rate Limiter/1 -> ograniczenie sygnalu/1
  ograniczenie sygnalu/1 -> dac_out/1

== system IRP/Const/Subsystem/serwo_4_5/serwo_5 ==
  wartosc_zad : Inport
  pomiar_poloz : Inport  Port=2
  Gain : Gain  Gain=0.5
  Rate Limiter : RateLimiter  RisingSlewLimit=50  FallingSlewLimit=-50  SampleTimeMode=inherited
  Saturation : Saturate  UpperLimit=3  LowerLimit=-3
  Sum : Sum  Inputs=|+-
  ograniczenie sygnalu : Gain  Gain=0.1
  dac_out : Outport
  wires:
  pomiar_poloz/1 -> Sum/2
  wartosc_zad/1 -> Sum/1
  Saturation/1 -> Rate Limiter/1
  Gain/1 -> Saturation/1
  Sum/1 -> Gain/1
  Rate Limiter/1 -> ograniczenie sygnalu/1
  ograniczenie sygnalu/1 -> dac_out/1

== system IRP/P /Position 1/Filters 1/Analog Butterworth LP Filter ==
  In1 : Inport
  Analog Butterworth LP Filter : ZeroPole  Zeros=z  Poles=p  Gain=k
  Out1 : Outport
  wires:
  In1/1 -> Analog Butterworth LP Filter/1
  Analog Butterworth LP Filter/1 -> Out1/1

== system IRP/P /Position 1/Filters 1/Analog Butterworth LP Filter1 ==
  In1 : Inport
  Analog Butterworth LP Filter1 : ZeroPole  Zeros=z  Poles=p  Gain=k
  Out1 : Outport
  wires:
  In1/1 -> Analog Butterworth LP Filter1/1
  Analog Butterworth LP Filter1/1 -> Out1/1

== system IRP/P /Position 2/Filters 2/Analog Butterworth LP Filter ==
  In1 : Inport
  Analog Butterworth LP Filter : ZeroPole  Zeros=z  Poles=p  Gain=k
  Out1 : Outport
  wires:
  In1/1 -> Analog Butterworth LP Filter/1
  Analog Butterworth LP Filter/1 -> Out1/1

== system IRP/P /Position 2/Filters 2/Analog Butterworth LP Filter1 ==
  In1 : Inport
  Analog Butterworth LP Filter1 : ZeroPole  Zeros=z  Poles=p  Gain=k
  Out1 : Outport
  wires:
  In1/1 -> Analog Butterworth LP Filter1/1
  Analog Butterworth LP Filter1/1 -> Out1/1

== system IRP/P /Position 3/Filters 3/Analog Butterworth LP Filter ==
  In1 : Inport
  Analog Butterworth LP Filter : ZeroPole  Zeros=z  Poles=p  Gain=k
  Out1 : Outport
  wires:
  In1/1 -> Analog Butterworth LP Filter/1
  Analog Butterworth LP Filter/1 -> Out1/1

== system IRP/P /Position 3/Filters 3/Analog Butterworth LP Filter1 ==
  In1 : Inport
  Analog Butterworth LP Filter1 : ZeroPole  Zeros=z  Poles=p  Gain=k
  Out1 : Outport
  wires:
  In1/1 -> Analog Butterworth LP Filter1/1
  Analog Butterworth LP Filter1/1 -> Out1/1

== system IRP/P /Position 4/Filters 4/Analog Butterworth LP Filter ==
  In1 : Inport
  Analog Butterworth LP Filter : ZeroPole  Zeros=z  Poles=p  Gain=k
  Out1 : Outport
  wires:
  In1/1 -> Analog Butterworth LP Filter/1
  Analog Butterworth LP Filter/1 -> Out1/1

== system IRP/P /Position 4/Filters 4/Analog Butterworth LP Filter1 ==
  In1 : Inport
  Analog Butterworth LP Filter1 : ZeroPole  Zeros=z  Poles=p  Gain=k
  Out1 : Outport
  wires:
  In1/1 -> Analog Butterworth LP Filter1/1
  Analog Butterworth LP Filter1/1 -> Out1/1

== system IRP/P /Position 5/Filters 5/Analog Butterworth LP Filter ==
  In1 : Inport
  Analog Butterworth LP Filter : ZeroPole  Zeros=z  Poles=p  Gain=k
  Out1 : Outport
  wires:
  In1/1 -> Analog Butterworth LP Filter/1
  Analog Butterworth LP Filter/1 -> Out1/1

== system IRP/P /Position 5/Filters 5/Analog Butterworth LP Filter1 ==
  In1 : Inport
  Analog Butterworth LP Filter1 : ZeroPole  Zeros=z  Poles=p  Gain=k
  Out1 : Outport
  wires:
  In1/1 -> Analog Butterworth LP Filter1/1
  Analog Butterworth LP Filter1/1 -> Out1/1

== system IRP/RTI Data/RTI Data Store/RTI Data Store/RTI Data Store ==
  RTI Data Store : Subsystem  mask(RTI_DATA_STORE){}
      mask help:
      | RTI Data Store Block. This block is used by RTI to store internal model dependent data. Deleting this block will result in data loss.
      |
      | NEVER DELETE, COPY, OR MODIFY THIS BLOCK!
      mask Help:
      | RTI Data Store Block. This block is used by RTI to store internal model dependent data. Deleting this block will result in data loss.
      | 
      | NEVER DELETE, COPY, OR MODIFY THIS BLOCK!
      mask Display: text(0.5, 0.5, ' ', 'HorizontalAlignment', 'center');

== system IRP/Const/Subsystem/Position 1/Filters 1/Analog Butterworth LP Filter ==
  In1 : Inport
  Analog Butterworth LP Filter : ZeroPole  Zeros=z  Poles=p  Gain=k
  Out1 : Outport
  wires:
  In1/1 -> Analog Butterworth LP Filter/1
  Analog Butterworth LP Filter/1 -> Out1/1

== system IRP/Const/Subsystem/Position 1/Filters 1/Analog Butterworth LP Filter1 ==
  In1 : Inport
  Analog Butterworth LP Filter1 : ZeroPole  Zeros=z  Poles=p  Gain=k
  Out1 : Outport
  wires:
  In1/1 -> Analog Butterworth LP Filter1/1
  Analog Butterworth LP Filter1/1 -> Out1/1

== system IRP/Const/Subsystem/Position 2/Filters 2/Analog Butterworth LP Filter ==
  In1 : Inport
  Analog Butterworth LP Filter : ZeroPole  Zeros=z  Poles=p  Gain=k
  Out1 : Outport
  wires:
  In1/1 -> Analog Butterworth LP Filter/1
  Analog Butterworth LP Filter/1 -> Out1/1

== system IRP/Const/Subsystem/Position 2/Filters 2/Analog Butterworth LP Filter1 ==
  In1 : Inport
  Analog Butterworth LP Filter1 : ZeroPole  Zeros=z  Poles=p  Gain=k
  Out1 : Outport
  wires:
  In1/1 -> Analog Butterworth LP Filter1/1
  Analog Butterworth LP Filter1/1 -> Out1/1

== system IRP/Const/Subsystem/Position 3/Filters 3/Analog Butterworth LP Filter ==
  In1 : Inport
  Analog Butterworth LP Filter : ZeroPole  Zeros=z  Poles=p  Gain=k
  Out1 : Outport
  wires:
  In1/1 -> Analog Butterworth LP Filter/1
  Analog Butterworth LP Filter/1 -> Out1/1

== system IRP/Const/Subsystem/Position 3/Filters 3/Analog Butterworth LP Filter1 ==
  In1 : Inport
  Analog Butterworth LP Filter1 : ZeroPole  Zeros=z  Poles=p  Gain=k
  Out1 : Outport
  wires:
  In1/1 -> Analog Butterworth LP Filter1/1
  Analog Butterworth LP Filter1/1 -> Out1/1

== system IRP/Const/Subsystem/serwo_4_5/Position 4/Filters 4 ==
  Sin && Cos : Inport
  Analog Butterworth LP Filter : Subsystem  mask(buttap){}
      mask help:
      | Analog Butterworth low pass filter.
      |
      | (Requires Signal Processing Toolbox)
      mask init:
      | [z,p,k]=buttap(@2); z=@1*z; p=@1*p; k=real(prod(-p)); [num,den]=zp2tf(z,p,k); w=logspace(log10(@1/10),log10(10*@1),20); h=freqs(num,den,w);
      mask Help: Butterworth low pass filter using MATLAB's butter command.
      mask Display: plot(20*log10(w),20*log10(abs(h)))
  Analog Butterworth LP Filter1 : Subsystem  mask(buttap){}
      mask help:
      | Analog Butterworth low pass filter.
      |
      | (Requires Signal Processing Toolbox)
      mask init:
      | [z,p,k]=buttap(@2); z=@1*z; p=@1*p; k=real(prod(-p)); [num,den]=zp2tf(z,p,k); w=logspace(log10(@1/10),log10(10*@1),20); h=freqs(num,den,w);
      mask Help: Butterworth low pass filter using MATLAB's butter command.
      mask Display: plot(20*log10(w),20*log10(abs(h)))
  Demux : Demux  Outputs=2
  Sin : Outport
  Cos : Outport  Port=2
  wires:
  Demux/2 -> Analog Butterworth LP Filter1/1(In1)
  Demux/1 -> Analog Butterworth LP Filter/1(In1)
  Sin && Cos/1 -> Demux/1
  Analog Butterworth LP Filter1/1(Out1) -> Cos/1
  Analog Butterworth LP Filter/1(Out1) -> Sin/1

== system IRP/Const/Subsystem/serwo_4_5/Position 4/Position Calculation 4 ==
  Sin : Inport
  Cos : Inport  Port=2
  Reset (Impulse) : Inport  Port=3
  Atan2 : Fcn  Expr=atan2(u[1],u[2])
  Conversion Rad to Deg : Gain  Gain=180/pi  SaturateOnIntegerOverflow=on  OutDataTypeStr=Inherit: Same as input  ParamDataTypeStr=Inherit: Same as input
  Conversion Rotation to Angle : Gain  Gain=2*pi  SaturateOnIntegerOverflow=on  OutDataTypeStr=Inherit: Same as input  ParamDataTypeStr=Inherit: Same as input
  Dead Zone : DeadZone  LowerValue=-5000  UpperValue=5000  SaturateOnIntegerOverflow=on
  Derivative : Derivative
  Gear : Gain  Gain=7.87e-3  SaturateOnIntegerOverflow=on  OutDataTypeStr=Inherit: Same as input  ParamDataTypeStr=Inherit: Same as input
  Init Angle : Switch  Threshold=1  SaturateOnIntegerOverflow=on  InputSameDT=on
  Memory : Memory
  Memory1 : Memory
  Mux : Mux  Inputs=2
  Product : Product  SaturateOnIntegerOverflow=on  RndMeth=Zero  InputSameDT=on  OutDataTypeStr=Inherit: Same as first input
  Saturation : Saturate  UpperLimit=1  LowerLimit=-1
  Sum : Sum  Inputs=+-  SaturateOnIntegerOverflow=on  InputSameDT=on  OutDataTypeStr=Inherit: Same as first input
  Sum1 : Sum  Inputs=++-  SaturateOnIntegerOverflow=on  InputSameDT=on  OutDataTypeStr=Inherit: Same as first input
  Position : Outport
  wires:
  Init Angle/1 -> Memory1/1, Sum1/3
  Memory1/1 -> Init Angle/1
  Product/1 -> Memory/1, Conversion Rotation to Angle/1
  Memory/1 -> Sum/1
  Cos/1 -> Mux/2
  Atan2/1 -> Init Angle/3, Sum1/2, Derivative/1
  Reset (Impulse)/1 -> Init Angle/2, Product/2
  Conversion Rotation to Angle/1 -> Sum1/1
  Saturation/1 -> Sum/2
  Conversion Rad to Deg/1 -> Position/1
  Sin/1 -> Mux/1
  Mux/1 -> Atan2/1
  Derivative/1 -> Dead Zone/1
  Dead Zone/1 -> Saturation/1
  Sum/1 -> Product/1
  Sum1/1 -> Gear/1
  Gear/1 -> Conversion Rad to Deg/1

== system IRP/Const/Subsystem/serwo_4_5/Position 5/Filters 5 ==
  Sin && Cos : Inport
  Analog Butterworth LP Filter : Subsystem  mask(buttap){}
      mask help:
      | Analog Butterworth low pass filter.
      |
      | (Requires Signal Processing Toolbox)
      mask init:
      | [z,p,k]=buttap(@2); z=@1*z; p=@1*p; k=real(prod(-p)); [num,den]=zp2tf(z,p,k); w=logspace(log10(@1/10),log10(10*@1),20); h=freqs(num,den,w);
      mask Help: Butterworth low pass filter using MATLAB's butter command.
      mask Display: plot(20*log10(w),20*log10(abs(h)))
  Analog Butterworth LP Filter1 : Subsystem  mask(buttap){}
      mask help:
      | Analog Butterworth low pass filter.
      |
      | (Requires Signal Processing Toolbox)
      mask init:
      | [z,p,k]=buttap(@2); z=@1*z; p=@1*p; k=real(prod(-p)); [num,den]=zp2tf(z,p,k); w=logspace(log10(@1/10),log10(10*@1),20); h=freqs(num,den,w);
      mask Help: Butterworth low pass filter using MATLAB's butter command.
      mask Display: plot(20*log10(w),20*log10(abs(h)))
  Demux : Demux  Outputs=2
  Sin : Outport
  Cos : Outport  Port=2
  wires:
  Demux/2 -> Analog Butterworth LP Filter1/1(In1)
  Demux/1 -> Analog Butterworth LP Filter/1(In1)
  Sin && Cos/1 -> Demux/1
  Analog Butterworth LP Filter1/1(Out1) -> Cos/1
  Analog Butterworth LP Filter/1(Out1) -> Sin/1

== system IRP/Const/Subsystem/serwo_4_5/Position 5/Position Calculation 5 ==
  Sin : Inport
  Cos : Inport  Port=2
  Reset (Impulse) : Inport  Port=3
  Atan2 : Fcn  Expr=atan2(u[1],u[2])
  Conversion Rad to Deg : Gain  Gain=180/pi  SaturateOnIntegerOverflow=on  OutDataTypeStr=Inherit: Same as input  ParamDataTypeStr=Inherit: Same as input
  Conversion Rotation to Angle : Gain  Gain=2*pi  SaturateOnIntegerOverflow=on  OutDataTypeStr=Inherit: Same as input  ParamDataTypeStr=Inherit: Same as input
  Dead Zone : DeadZone  LowerValue=-5000  UpperValue=5000  SaturateOnIntegerOverflow=on
  Derivative : Derivative
  Gear : Gain  Gain=1.32e-2  SaturateOnIntegerOverflow=on  OutDataTypeStr=Inherit: Same as input  ParamDataTypeStr=Inherit: Same as input
  Init Angle : Switch  Threshold=1  SaturateOnIntegerOverflow=on  InputSameDT=on
  Memory : Memory
  Memory1 : Memory
  Mux : Mux  Inputs=2
  Product : Product  SaturateOnIntegerOverflow=on  RndMeth=Zero  InputSameDT=on  OutDataTypeStr=Inherit: Same as first input
  Saturation : Saturate  UpperLimit=1  LowerLimit=-1
  Sum : Sum  Inputs=+-  SaturateOnIntegerOverflow=on  InputSameDT=on  OutDataTypeStr=Inherit: Same as first input
  Sum1 : Sum  Inputs=++-  SaturateOnIntegerOverflow=on  InputSameDT=on  OutDataTypeStr=Inherit: Same as first input
  Position : Outport
  wires:
  Init Angle/1 -> Memory1/1, Sum1/3
  Memory1/1 -> Init Angle/1
  Product/1 -> Memory/1, Conversion Rotation to Angle/1
  Memory/1 -> Sum/1
  Cos/1 -> Mux/2
  Atan2/1 -> Init Angle/3, Sum1/2, Derivative/1
  Reset (Impulse)/1 -> Init Angle/2, Product/2
  Conversion Rotation to Angle/1 -> Sum1/1
  Saturation/1 -> Sum/2
  Conversion Rad to Deg/1 -> Position/1
  Sin/1 -> Mux/1
  Mux/1 -> Atan2/1
  Derivative/1 -> Dead Zone/1
  Dead Zone/1 -> Saturation/1
  Sum/1 -> Product/1
  Sum1/1 -> Gear/1
  Gear/1 -> Conversion Rad to Deg/1

== system IRP/RTI Data/RTI Data Store/RTI Data Store/RTI Data Store/RTI Data Store ==

== system IRP/Const/Subsystem/serwo_4_5/Position 4/Filters 4/Analog Butterworth LP Filter ==
  In1 : Inport
  Analog Butterworth LP Filter : ZeroPole  Zeros=z  Poles=p  Gain=k
  Out1 : Outport
  wires:
  In1/1 -> Analog Butterworth LP Filter/1
  Analog Butterworth LP Filter/1 -> Out1/1

== system IRP/Const/Subsystem/serwo_4_5/Position 4/Filters 4/Analog Butterworth LP Filter1 ==
  In1 : Inport
  Analog Butterworth LP Filter1 : ZeroPole  Zeros=z  Poles=p  Gain=k
  Out1 : Outport
  wires:
  In1/1 -> Analog Butterworth LP Filter1/1
  Analog Butterworth LP Filter1/1 -> Out1/1

== system IRP/Const/Subsystem/serwo_4_5/Position 5/Filters 5/Analog Butterworth LP Filter ==
  In1 : Inport
  Analog Butterworth LP Filter : ZeroPole  Zeros=z  Poles=p  Gain=k
  Out1 : Outport
  wires:
  In1/1 -> Analog Butterworth LP Filter/1
  Analog Butterworth LP Filter/1 -> Out1/1

== system IRP/Const/Subsystem/serwo_4_5/Position 5/Filters 5/Analog Butterworth LP Filter1 ==
  In1 : Inport
  Analog Butterworth LP Filter1 : ZeroPole  Zeros=z  Poles=p  Gain=k
  Out1 : Outport
  wires:
  In1/1 -> Analog Butterworth LP Filter1/1
  Analog Butterworth LP Filter1/1 -> Out1/1
